simulink model "schem_3"  (R2024a)
settings: Solver=VariableStepAuto  StartTime=0.0  StopTime=100  RelTol=1e-3
undefined symbols (not defined in the file): G1, G2, xi20
settings Model: Creator=user  LastModifiedBy=user

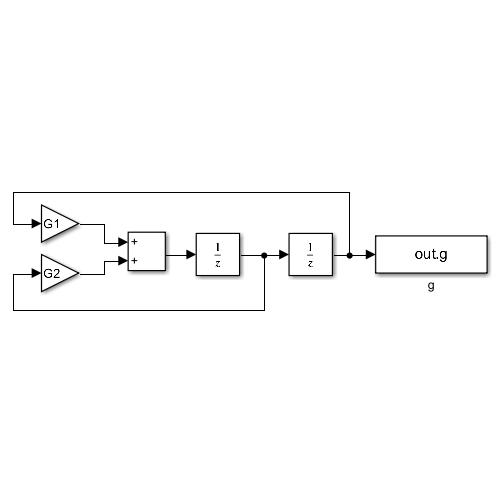
[thumbnail: Simulink's stored preview of the top-level diagram]
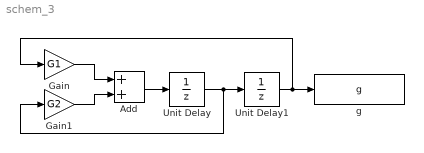
== system schem_3 ==
  Add : Sum
  Gain : Gain  Gain=G1
  Gain1 : Gain  Gain=G2
  Unit Delay : UnitDelay  InitialCondition=xi20  SampleTime=0.2  HasFrameUpgradeWarning=on
  Unit Delay1 : UnitDelay  SampleTime=0.2  HasFrameUpgradeWarning=on
  g : ToWorkspace  VariableName=g  SaveFormat=Timeseries  SampleTime=-1
  wires:
  Add/1 -> Unit Delay/1
  Gain1/1 -> Add/2
  Unit Delay/1 -> Gain1/1, Unit Delay1/1
  Unit Delay1/1 -> g/1, Gain/1
  Gain/1 -> Add/1
